simulink model "test_getConnectedSegments"  (R2017a)
settings: Solver=VariableStepAuto  StartTime=0.0  StopTime=10.0  RelTol=1e-3
settings Model: Creator=GM  LastModifiedBy=GM

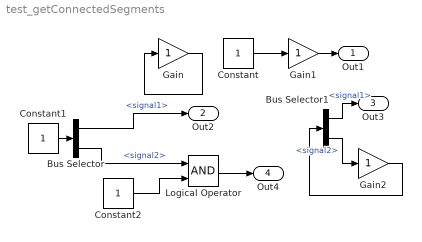
== system test_getConnectedSegments ==
  Bus Selector : BusSelector  OutputSignals=signal1,signal2
  Bus Selector1 : BusSelector  OutputSignals=signal1,signal2
  Constant : Constant
  Constant1 : Constant
  Constant2 : Constant
  Gain : Gain
  Gain1 : Gain
  Gain2 : Gain
  Logical Operator : Logic  AllPortsSameDT=off  OutDataTypeStr=boolean
  Out1 : Outport
  Out2 : Outport  Port=2
  Out3 : Outport  Port=3
  Out4 : Outport  Port=4
  wires:
  Gain/1 -> Gain/1
  Constant/1 -> Gain1/1
  Gain1/1 -> Out1/1
  Bus Selector/2 -> Logical Operator/1  "<signal2>"
  Bus Selector/1 -> Out2/1  "<signal1>"
  Constant1/1 -> Bus Selector/1
  Constant2/1 -> Logical Operator/2
  Logical Operator/1 -> Out4/1
  Bus Selector1/1 -> Out3/1  "<signal1>"
  Bus Selector1/2 -> Gain2/1  "<signal2>"
  Gain2/1 -> Bus Selector1/1
